simulink model "motion_of_a_vacuum_cleaner"  (R2019b)
settings: Solver=VariableStepAuto  StartTime=0.0  StopTime=20  RelTol=1e-3
undefined symbols (not defined in the file): m, magnitude, r
libraries: simulink x1
settings Model: Creator=46769  LastModifiedBy=chiragg
settings DebuggingCC: SFMachineParentedDataDiag=error

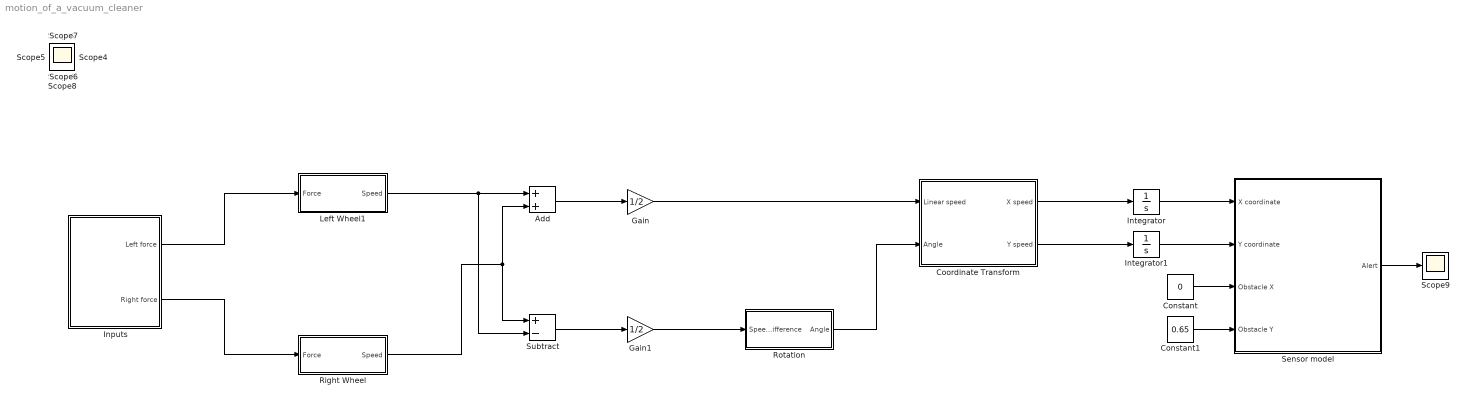
== system motion_of_a_vacuum_cleaner ==
  Add : Sum
  Constant : Constant  Value=0
  Constant1 : Constant  Value=0.65
  Coordinate Transform : Subsystem
  Gain : Gain  Gain=1/2
  Gain1 : Gain  Gain=1/2
  Inputs : Subsystem
  Integrator : Integrator
  Integrator1 : Integrator
  Left Wheel1 : Subsystem
  Right Wheel : Subsystem
  Rotation : Subsystem
  Scope{1..9} (9 alike) : Scope
  "Sensor model " : Subsystem
  Subtract : Sum  Inputs=+-
  wires:
  Left Wheel1/1(Speed) -> Subtract/2, Add/1
  Right Wheel/1(Speed) -> Subtract/1, Add/2
  Add/1 -> Gain/1
  Subtract/1 -> Gain1/1
  Gain/1 -> Coordinate Transform/1(Linear speed)
  Gain1/1 -> Rotation/1(Speed difference)
  Rotation/1(Angle) -> Coordinate Transform/2(Angle)
  Coordinate Transform/1(X speed) -> Integrator/1
  Coordinate Transform/2(Y speed) -> Integrator1/1
  Inputs/1(Left force) -> Left Wheel1/1(Force)
  Inputs/2(Right force) -> Right Wheel/1(Force)
  Integrator1/1 -> "Sensor model "/2(Y coordinate)
  Integrator/1 -> "Sensor model "/1(X coordinate)
  Constant1/1 -> "Sensor model "/4("Obstacle Y ")
  Constant/1 -> "Sensor model "/3(Obstacle X)
  "Sensor model "/1("Alert ") -> Scope9/1

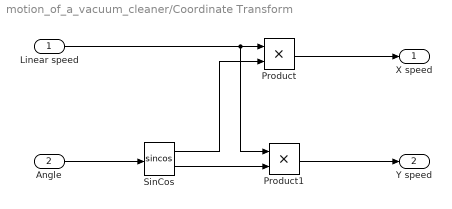
== system motion_of_a_vacuum_cleaner/Coordinate Transform ==
  Linear speed : Inport
  Angle : Inport  Port=2
  Product : Product
  Product1 : Product
  SinCos : Trigonometry  Operator=sincos
  X speed : Outport
  Y speed : Outport  Port=2
  wires:
  Angle/1 -> SinCos/1
  Linear speed/1 -> Product1/1, Product/1
  SinCos/1 -> Product/2
  SinCos/2 -> Product1/2
  Product/1 -> X speed/1
  Product1/1 -> Y speed/1

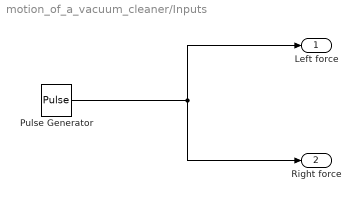
== system motion_of_a_vacuum_cleaner/Inputs ==
  Pulse Generator : DiscretePulseGenerator  PulseType=Time based  Period=20  PulseWidth=15
  Left force : Outport
  Right force : Outport  Port=2
  wires:
  Pulse Generator/1 -> Left force/1, Right force/1

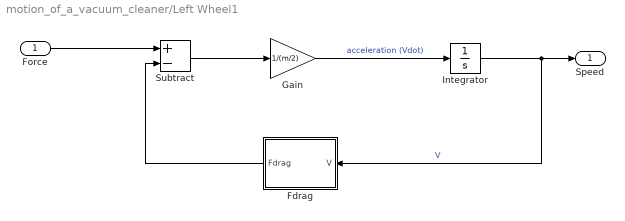
== system motion_of_a_vacuum_cleaner/Left Wheel1 ==
  Force : Inport
  Fdrag : MATLAB Function  TreatAsAtomicUnit=on
  Gain : Gain  Gain=1/(m/2)
  Integrator : Integrator
  Subtract : Sum  Inputs=+-
  Speed : Outport
  wires:
  Gain/1 -> Integrator/1  "acceleration (Vdot)"
  Subtract/1 -> Gain/1
  Fdrag/1(Fdrag) -> Subtract/2
  Force/1 -> Subtract/1
  Integrator/1 -> Speed/1, Fdrag/1(V)  "V"

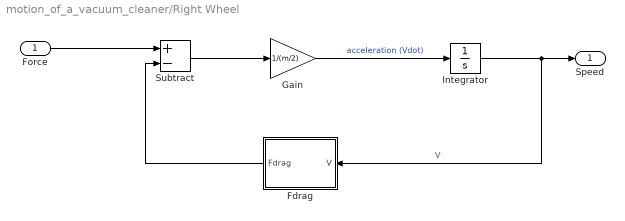
== system motion_of_a_vacuum_cleaner/Right Wheel ==
  Force : Inport
  Fdrag : MATLAB Function  TreatAsAtomicUnit=on
  Gain : Gain  Gain=1/(m/2)
  Integrator : Integrator
  Subtract : Sum  Inputs=+-
  Speed : Outport
  wires:
  Integrator/1 -> Fdrag/1(V), Speed/1  "V"
  Force/1 -> Subtract/1
  Fdrag/1(Fdrag) -> Subtract/2
  Subtract/1 -> Gain/1
  Gain/1 -> Integrator/1  "acceleration (Vdot)"

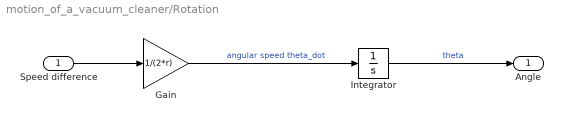
== system motion_of_a_vacuum_cleaner/Rotation ==
  Speed difference : Inport
  Gain : Gain  Gain=1/(2*r)
  Integrator : Integrator
  Angle : Outport
  wires:
  Speed difference/1 -> Gain/1
  Gain/1 -> Integrator/1  "angular speed theta_dot"
  Integrator/1 -> Angle/1  "theta"

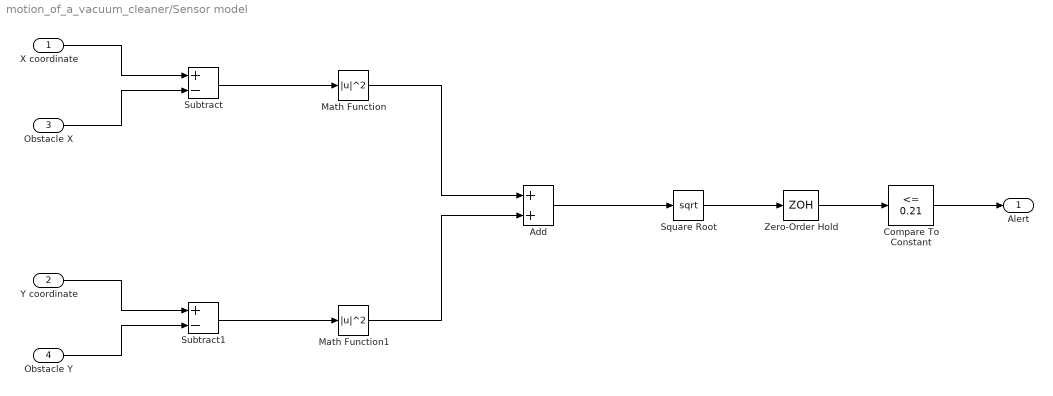
== system motion_of_a_vacuum_cleaner/Sensor model  ==
  X coordinate : Inport
  Y coordinate : Inport  Port=2
  Obstacle X : Inport  Port=3
  "Obstacle Y " : Inport  Port=4
  Add : Sum
  Compare To Constant : simulink/Logic and Bit Operations/Compare To Constant  relop=<=  const=0.21  OutDataTypeStr=boolean
  Math Function : Math  Operator=magnitude^2  SignedPower=off  SaturateOnIntegerOverflow=on
  Math Function1 : Math  Operator=magnitude^2  SignedPower=off  SaturateOnIntegerOverflow=on
  Square Root : Sqrt  SaturateOnIntegerOverflow=on
  Subtract : Sum  Inputs=+-
  Subtract1 : Sum  Inputs=+-
  Zero-Order Hold : ZeroOrderHold  SampleTime=0.25
  "Alert " : Outport
  wires:
  X coordinate/1 -> Subtract/1
  Obstacle X/1 -> Subtract/2
  Y coordinate/1 -> Subtract1/1
  "Obstacle Y "/1 -> Subtract1/2
  Subtract/1 -> Math Function/1
  Subtract1/1 -> Math Function1/1
  Math Function/1 -> Add/1
  Math Function1/1 -> Add/2
  Add/1 -> Square Root/1
  Square Root/1 -> Zero-Order Hold/1
  Zero-Order Hold/1 -> Compare To Constant/1
  Compare To Constant/1 -> "Alert "/1

== matlab function motion_of_a_vacuum_cleaner/Left Wheel1/Fdrag ==
  data: V input; Fdrag output; k_drag parameter
function Fdrag = get_fdrag(V, k_drag)

Fdrag = k_drag*V*abs(V);

== matlab function motion_of_a_vacuum_cleaner/Right Wheel/Fdrag ==
  data: V input; Fdrag output; k_drag parameter
function Fdrag = get_fdrag(V, k_drag)

Fdrag = k_drag*V*abs(V);
